simulink model "dp_real_vs_lin"  (R2015b)
settings: Solver=VariableStepAuto  StartTime=0.0  StopTime=10  FixedStep=T_s  RelTol=1e-3
InitFcn:
  | dp_real_vs_lin_script
values from neighbouring files (symbols this model uses):
  A6 = [0 1 0 0 0 0 ... (first row only)    [dp_EKF_script.m]    (also in dp_kalman_script.m; dp_real_vs_lin_script.m; dp_statefeedback_script.m)
  Ad6 = sys6d.a    [dp_EKF_script.m]    (also in dp_kalman_script.m; dp_real_vs_lin_script.m; dp_statefeedback_script.m)
  B6 = [0;1; 0; b2; 0; b4]    [dp_EKF_script.m]    (also in dp_kalman_script.m; dp_real_vs_lin_script.m; dp_statefeedback_script.m)
  Bd6 = sys6d.b    [dp_EKF_script.m]    (also in dp_kalman_script.m; dp_real_vs_lin_script.m; dp_statefeedback_script.m)
  C6 = [1 0 0 0 0 0 ... (first row only)    [dp_EKF_script.m]    (also in dp_kalman_script.m; dp_real_vs_lin_script.m; dp_statefeedback_script.m)
  Cd6 = sys6d.c    [dp_EKF_script.m]    (also in dp_kalman_script.m; dp_real_vs_lin_script.m; dp_statefeedback_script.m)
  D6 = [0;0;0;]    [dp_EKF_script.m]    (also in dp_kalman_script.m; dp_real_vs_lin_script.m; dp_statefeedback_script.m)
  d_p1 = 0.001    [dp_EKF_script.m]    (also in dp_UKF_script.m; dp_kalman_script.m; dp_real_vs_lin_script.m; dp_statefeedback_script.m)
  d_p2 = 0.001    [dp_EKF_script.m]    (also in dp_UKF_script.m; dp_kalman_script.m; dp_real_vs_lin_script.m; dp_statefeedback_script.m)
  g = 9.81    [dp_EKF_script.m]    (also in dp_UKF_script.m; dp_kalman_script.m; dp_real_vs_lin_script.m; dp_statefeedback_script.m)
  l_1 = 0.194    [dp_EKF_script.m]    (also in dp_UKF_script.m; dp_kalman_script.m; dp_real_vs_lin_script.m; dp_statefeedback_script.m)
  l_2 = 0.1855    [dp_EKF_script.m]    (also in dp_UKF_script.m; dp_kalman_script.m; dp_real_vs_lin_script.m; dp_statefeedback_script.m)
  m_1 = 0.0313    [dp_EKF_script.m]    (also in dp_UKF_script.m; dp_kalman_script.m; dp_real_vs_lin_script.m; dp_statefeedback_script.m)
  m_2 = 0.0313    [dp_EKF_script.m]    (also in dp_UKF_script.m; dp_kalman_script.m; dp_real_vs_lin_script.m; dp_statefeedback_script.m)
  m_3 = 0.0308    [dp_EKF_script.m]    (also in dp_UKF_script.m; dp_kalman_script.m; dp_real_vs_lin_script.m; dp_statefeedback_script.m)
  T_s = 0.001    [dp_EKF_script.m]    (also in dp_UKF_script.m; dp_kalman_script.m; dp_real_vs_lin_script.m; dp_statefeedback_script.m)
  x0_6 = [x_0; dx_0; phi1_0; dphi1_0; phi2_0; dphi2_0]    [dp_real_vs_lin_script.m]
undefined symbols (not defined in the file or in its folder): K6_lqr
libraries: simulink x3
settings Model: Creator=serov  LastModifiedBy=serov

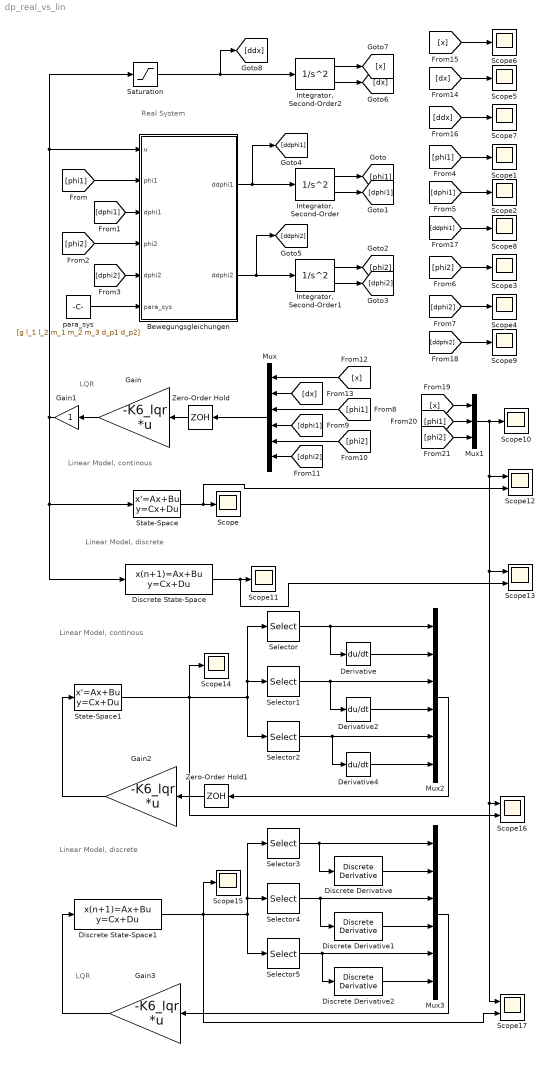
== system dp_real_vs_lin ==
  note: LQR
  note: Real System
  note: Linear Model, discrete
  note: Linear Model, continous
  note: Linear Model, continous
  note: Linear Model, discrete
  note: LQR
  Bewegungsgleichungen : MATLAB Function  TreatAsAtomicUnit=on
  Derivative : Derivative
  Derivative2 : Derivative
  Derivative4 : Derivative
  Discrete Derivative : simulink/Discrete/Discrete Derivative  gainval=1.0  ICPrevScaledInput=0.0  InputProcessing=Inherited  OutMin=[]  OutMax=[]  OutDataType=fixdt(1, 16)  OutScaling=2^-10  DoSatur=off
  Discrete Derivative1 : simulink/Discrete/Discrete Derivative  gainval=1.0  ICPrevScaledInput=0.0  InputProcessing=Inherited  OutMin=[]  OutMax=[]  OutDataType=fixdt(1, 16)  OutScaling=2^-10  DoSatur=off
  Discrete Derivative2 : simulink/Discrete/Discrete Derivative  gainval=1.0  ICPrevScaledInput=0.0  InputProcessing=Inherited  OutMin=[]  OutMax=[]  OutDataType=fixdt(1, 16)  OutScaling=2^-10  DoSatur=off
  Discrete State-Space : DiscreteStateSpace  A=Ad6  B=Bd6  C=Cd6  D=D6  X0=x0_6  SampleTime=T_s
  Discrete State-Space1 : DiscreteStateSpace  A=Ad6  B=Bd6  C=Cd6  D=D6  X0=x0_6  SampleTime=T_s
  Gain : Gain  Gain=-K6_lqr  Multiplication=Matrix(K*u) (u vector)
  Gain1 : Gain
  Gain2 : Gain  Gain=-K6_lqr  Multiplication=Matrix(K*u) (u vector)
  Gain3 : Gain  Gain=-K6_lqr  Multiplication=Matrix(K*u) (u vector)
  "Integrator, Second-Order" : SecondOrderIntegrator  ICX=phi1_0  ICDXDT=dphi1_0
  "Integrator, Second-Order1" : SecondOrderIntegrator  ICX=phi2_0  ICDXDT=dphi2_0
  "Integrator, Second-Order2" : SecondOrderIntegrator  ICX=x_0  LimitX=on  UpperLimitX=0.2  LowerLimitX=-0.2  ICDXDT=dx_0  LimitDXDT=on  UpperLimitDXDT=5  LowerLimitDXDT=-5
  Mux : Mux  Inputs=6
  Mux1 : Mux  Inputs=3
  Mux2 : Mux  Inputs=6
  Mux3 : Mux  Inputs=6
  Saturation : Saturate  UpperLimit=20  LowerLimit=-20
  Scope{,1..11,14..15} (14 alike) : Scope
  Scope{12..13,16..17} (4 alike) : Scope  NumInputPorts=2
  Selector : Selector  InputPortWidth=3  IndexOptions=Index vector (dialog)  Indices=[1]  OutputSizes=1
  Selector1 : Selector  InputPortWidth=3  IndexOptions=Index vector (dialog)  Indices=[2]  OutputSizes=1
  Selector2 : Selector  InputPortWidth=3  IndexOptions=Index vector (dialog)  Indices=[3]  OutputSizes=1
  Selector3 : Selector  InputPortWidth=3  IndexOptions=Index vector (dialog)  Indices=[1]  OutputSizes=1
  Selector4 : Selector  InputPortWidth=3  IndexOptions=Index vector (dialog)  Indices=[2]  OutputSizes=1
  Selector5 : Selector  InputPortWidth=3  IndexOptions=Index vector (dialog)  Indices=[3]  OutputSizes=1
  State-Space : StateSpace  A=A6  B=B6  C=C6  D=D6  X0=x0_6
  State-Space1 : StateSpace  A=A6  B=B6  C=C6  D=D6  X0=x0_6
  Zero-Order Hold : ZeroOrderHold  SampleTime=T_s
  Zero-Order Hold1 : ZeroOrderHold  SampleTime=T_s
  para_sys : Constant  Value=[g l_1 l_2 m_1 m_2 m_3 d_p1 d_p2]
  wires:
  Bewegungsgleichungen/1(ddphi1) -> [ddphi1], "Integrator, Second-Order"/1
  Bewegungsgleichungen/2(ddphi2) -> [ddphi2], "Integrator, Second-Order1"/1
  "Integrator, Second-Order"/1 -> [phi1]
  "Integrator, Second-Order"/2 -> [dphi1]
  "Integrator, Second-Order1"/2 -> [dphi2]
  "Integrator, Second-Order1"/1 -> [phi2]
  [phi1] -> Bewegungsgleichungen/2(phi1)
  [dphi1] -> Bewegungsgleichungen/3(dphi1)
  [phi2] -> Bewegungsgleichungen/4(phi2)
  [dphi2] -> Bewegungsgleichungen/5(dphi2)
  para_sys/1 -> Bewegungsgleichungen/6(para_sys)
  [phi1] -> Scope1/1
  [dphi1] -> Scope2/1
  [phi2] -> Scope3/1
  [dphi2] -> Scope4/1
  [phi1] -> Mux/3
  [dphi1] -> Mux/4
  [phi2] -> Mux/5
  [dphi2] -> Mux/6
  Mux/1 -> Zero-Order Hold/1
  "Integrator, Second-Order2"/1 -> [x]
  "Integrator, Second-Order2"/2 -> [dx]
  [x] -> Mux/1
  [dx] -> Mux/2
  [dx] -> Scope5/1
  [x] -> Scope6/1
  [ddx] -> Scope7/1
  [ddphi1] -> Scope8/1
  [ddphi2] -> Scope9/1
  Saturation/1 -> [ddx], "Integrator, Second-Order2"/1
  [x] -> Mux1/1
  [phi1] -> Mux1/2
  [phi2] -> Mux1/3
  Zero-Order Hold/1 -> Gain/1
  State-Space/1 -> Scope12/2, Scope/1
  Discrete State-Space/1 -> Scope13/2, Scope11/1
  Gain1/1 -> Discrete State-Space/1, State-Space/1, Saturation/1, Bewegungsgleichungen/1(u)
  Gain/1 -> Gain1/1
  Mux1/1 -> Scope17/1, Scope16/1, Scope13/1, Scope12/1, Scope10/1
  State-Space1/1 -> Scope16/2, Selector1/1, Selector/1, Selector2/1, Scope14/1
  Selector/1 -> Mux2/1, Derivative/1
  Selector1/1 -> Mux2/3, Derivative2/1
  Selector2/1 -> Mux2/5, Derivative4/1
  Mux2/1 -> Zero-Order Hold1/1
  Zero-Order Hold1/1 -> Gain2/1
  Gain2/1 -> State-Space1/1
  Derivative/1 -> Mux2/2
  Derivative2/1 -> Mux2/4
  Derivative4/1 -> Mux2/6
  Discrete State-Space1/1 -> Scope17/2, Selector4/1, Selector3/1, Selector5/1, Scope15/1
  Selector3/1 -> Mux3/1, Discrete Derivative/1
  Selector4/1 -> Discrete Derivative1/1, Mux3/3
  Selector5/1 -> Discrete Derivative2/1, Mux3/5
  Mux3/1 -> Gain3/1
  Gain3/1 -> Discrete State-Space1/1
  Discrete Derivative/1 -> Mux3/2
  Discrete Derivative1/1 -> Mux3/4
  Discrete Derivative2/1 -> Mux3/6

== matlab function dp_real_vs_lin/Bewegungsgleichungen ==
  data: u input; phi1 input; dphi1 input; phi2 input; dphi2 input; para_sys input; ddphi1 output; ddphi2 output
function [ddphi1, ddphi2] = pendel_1_2(u, phi1, dphi1, phi2, dphi2, para_sys)
%#codegen

g = para_sys(1);
l_1 = para_sys(2);
l_2 = para_sys(3);
m_1 = para_sys(4);
m_2 = para_sys(5);
m_3 = para_sys(6);
d_p1 = para_sys(7);
d_p2 = para_sys(8);

ddphi1 = 1/(l_1^2*(9*cos(phi1-phi2)^2*m_2-4*m_1-12*m_2-12*m_3)*l_2)*(9*dphi1^2*cos(phi1-phi2)*sin(phi1-phi2)*l_1^2*l_2*m_2+6*m_2*l_1*l_2^2*sin(phi1-phi2)*dphi2^2+9*u*cos(phi1-phi2)*cos(phi2)*l_1*l_2*m_2+9*cos(phi1-phi2)*sin(phi2)*g*l_1*l_2*m_2-6*l_1*cos(phi1)*u*m_1*l_2-12*l_1*cos(phi1)*u*m_2*l_2-12*l_1*cos(phi1)*u*m_3*l_2-6*l_1*g*sin(phi1)*m_1*l_2-12*l_1*g*sin(phi1)*m_2*l_2-12*l_1*g*sin(phi1)*m_3*l_2+18*dphi1*cos(phi1-phi2)*d_p2*l_1-18*dphi2*cos(phi1-phi2)*d_p2*l_1+12*dphi1*d_p1*l_2+12*dphi1*d_p2*l_2-12*d_p2*dphi2*l_2);

ddphi2 = -1/(l_1*l_2^2*(9*cos(phi1-phi2)^2*m_2-4*m_1-12*m_2-12*m_3)*m_2)*(12*dphi1*d_p2*l_1*m_1+36*dphi1*d_p2*l_1*m_2+36*dphi1*d_p2*l_1*m_3-12*dphi2*d_p2*l_1*m_1-36*dphi2*d_p2*l_1*m_2-36*dphi2*d_p2*l_1*m_3-9*cos(phi1)*u*cos(phi1-phi2)*l_1*l_2*m_1*m_2-18*cos(phi1)*u*cos(phi1-phi2)*l_1*l_2*m_2*m_3-9*cos(phi1-phi2)*sin(phi1)*g*l_1*l_2*m_1*m_2-18*cos(phi1-phi2)*sin(phi1)*g*l_1*l_2*m_2*m_3+9*dphi2^2*cos(phi1-phi2)*sin(phi1-phi2)*l_1*l_2^2*m_2^2+ 6*dphi1^2*sin(phi1-phi2)*l_1^2*l_2*m_1*m_2+ 18*dphi1^2*sin(phi1-phi2)*l_1^2*l_2*m_2*m_3-18*cos(phi1)*u*cos(phi1-phi2)*l_1*l_2*m_2^2-18*cos(phi1-phi2)*sin(phi1)*g*l_1*l_2*m_2^2 +6*u*cos(phi2)*l_1*l_2*m_1*m_2+18*u*cos(phi2)*l_1*l_2*m_2*m_3+6*sin(phi2)*g*l_1*l_2*m_1*m_2+18*sin(phi2)*g*l_1*l_2*m_2*m_3 + 18*(dphi1)^2*sin(phi1-phi2)*l_1^2*l_2*m_2^2+18*u*cos(phi2)*l_1*l_2*m_2^2+18*sin(phi2)*g*l_1*l_2*m_2^2+18*dphi1*cos(phi1-phi2)*d_p1*l_2*m_2 + 18*dphi1*cos(phi1-phi2)*d_p2*l_2*m_2-18*dphi2*cos(phi1-phi2)*d_p2*l_2*m_2);
